simulink model "Output_Feedback"  (R2022b)
settings: Solver=FixedStepAuto  StartTime=0.0  StopTime=10.0  FixedStep=step_size  RelTol=1e-3
undefined symbols (not defined in the file): b, k1, k2, theta_i, x_i, y_i
libraries: simulink_extras x1
settings Model: Creator=Musta  LastModifiedBy=Musta

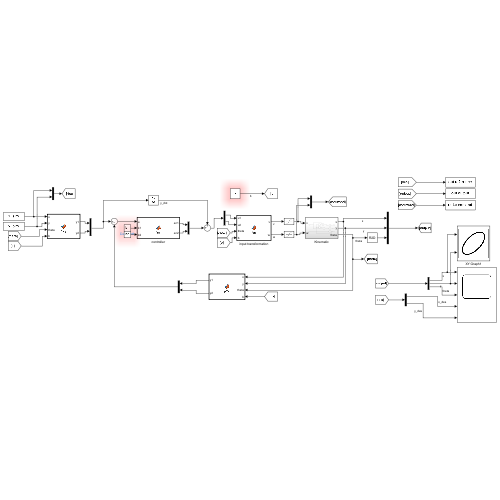
[thumbnail: Simulink's stored preview of the top-level diagram]
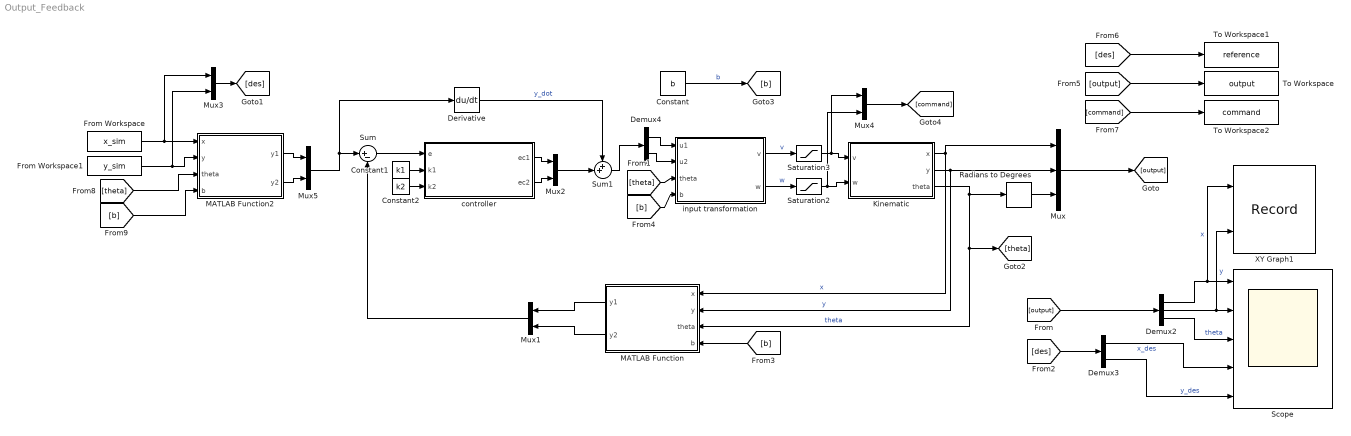
== system Output_Feedback ==
  Constant : Constant  Value=b
  Constant1 : Constant  Value=k1
  Constant2 : Constant  Value=k2
  Demux2 : Demux  Outputs=3
  Demux3 : Demux  Outputs=2
  Demux4 : Demux  Outputs=2
  Derivative : Derivative
  From Workspace : FromWorkspace  VariableName=x_sim
  From Workspace1 : FromWorkspace  VariableName=y_sim
  Kinematic : Subsystem
  MATLAB Function : MATLAB Function  TreatAsAtomicUnit=on
  MATLAB Function2 : MATLAB Function  TreatAsAtomicUnit=on
  Mux : Mux  Inputs=3
  Mux{1..5} (5 alike) : Mux  Inputs=2
  Radians to Degrees : simulink_extras/Transformations/Radians to Degrees
  Saturation2 : Saturate  UpperLimit=2  LowerLimit=-2
  Saturation3 : Saturate  UpperLimit=2  LowerLimit=-2
  Scope : Scope  NumInputPorts=5
  Sum : Sum  Inputs=|+-
  Sum1 : Sum  Inputs=++|
  To Workspace : ToWorkspace  VariableName=output  SaveFormat=Structure With Time  SampleTime=-1
  To Workspace1 : ToWorkspace  VariableName=reference  SaveFormat=Structure With Time  SampleTime=-1
  To Workspace2 : ToWorkspace  VariableName=command  SaveFormat=Structure With Time  SampleTime=-1
  XY Graph1 : Record  FileSettingsInternal="{\"entries\":[{\"content\":{\"excelSettings\":{\"content\":{},\"type\":\"Streamout.ExcelSettings\"}},\"type\":\"Streamout.FileSettingStorage\",\"uuid\":\"0d4e8405-cc65-47cc-850f-a12000fc69a0\"}],\"packageUris\":[\"http://schema.mathworks.com/mf0/streamout_blocks/R2020a\"],\"version\":\"1.0\"}"  Layout=[1 1]  SignalsInternal="{\"entries\":[{\"content\":{\"signals\":[{\"content\":{\"blockPath\":[\"Output_Feedback_MATLAB/XY Graph1\"],\"channel\":[],\"dimensions\":[1],\"domain\":\"Output_Feedback_MATLAB/XY Graph1\",\"lineColor\":\"#a2142f\",\"plots\":[1],\"port\":1,\"sid\":[\"\"],\"signalID\":860,\"signalName\":\"x\"},\"type\":\"RecordBlkView.Signal\",\"uuid\":\"881d64ae-a7b1-402c-b34c-8b1dce287662\"},{\"content\":{\"blockPath\":[\"Output_Feedback_MATLAB/XY Graph1\"],\"channel\":[],\"dimensions\":[1],\"domain\":\"Output_Feedback_MATLAB/XY Graph1\",\"lineColor\":\"#139fff\",\"plots\":[1],\"port\":2,\"sid\":[\"\"],\"signalID\":864,\"signalName\":\"y\"},\"type\":\"RecordBlkView.Signal\",\"uuid\":\"d56edbe0-4863-4ce2-984c-3d6a7468b7cc\"}]},\"type\":\"RecordBlkView.InputSignals\",\"uuid\":\"a5a01336-52e2-4cfc-b20a-f4ad49d08ddd\"}],\"packageUris\":[\"http://schema.mathworks.com/mf0/streamout_blocks/R2020a\"],\"version\":\"1.0\"}"  VisualizationBindings="{\"xyplotplugin\":{\"info\":[{\"series\":[{\"bindingParametersList\":[{\"parameter\":\"X-Axis\",\"signalID\":860,\"signalName\":\"x\"},{\"parameter\":\"Y-Axis\",\"signalID\":864,\"signalName\":\"y\"}],\"seriesID\":40151}],\"subplotID\":1}]}}"  CompatibilityTag=XY
  controller : MATLAB Function  TreatAsAtomicUnit=on
  input transformation : MATLAB Function  TreatAsAtomicUnit=on
  wires:
  [command] -> To Workspace2/1
  Mux4/1 -> [command]
  From Workspace/1 -> Mux3/1, MATLAB Function2/1(x)
  Mux3/1 -> [des]
  [theta] -> MATLAB Function2/3(theta)
  Mux1/1 -> Sum/2
  Radians to Degrees/1 -> Mux/3
  From Workspace1/1 -> Mux3/2, MATLAB Function2/2(y)
  MATLAB Function2/2(y2) -> Mux5/2
  Saturation3/1 -> Kinematic/1(v), Mux4/1
  [des] -> To Workspace1/1
  [des] -> Demux3/1
  [b] -> MATLAB Function/4(b)
  MATLAB Function/2(y2) -> Mux1/2
  MATLAB Function2/1(y1) -> Mux5/1
  [b] -> MATLAB Function2/4(b)
  Derivative/1 -> Sum1/1  "y_dot"
  Mux/1 -> [output]
  Mux5/1 -> Derivative/1, Sum/1
  Demux4/1 -> input transformation/1(u1)
  [theta] -> input transformation/3(theta)
  [output] -> To Workspace/1
  Sum/1 -> controller/1(e)
  Demux4/2 -> input transformation/2(u2)
  Demux2/2 -> XY Graph1/2, Scope/2  "y"
  controller/1(ec1) -> Mux2/1
  [output] -> Demux2/1
  Mux2/1 -> Sum1/2
  Demux2/3 -> Scope/3  "theta"
  Demux3/2 -> Scope/5  "y_des"
  input transformation/1(v) -> Saturation3/1  "v"
  Saturation2/1 -> Kinematic/2(w), Mux4/2
  Constant/1 -> [b]  "b"
  Sum1/1 -> Demux4/1
  Demux2/1 -> XY Graph1/1, Scope/1  "x"
  controller/2(ec2) -> Mux2/2
  MATLAB Function/1(y1) -> Mux1/1
  [b] -> input transformation/4(b)
  Kinematic/3(theta) -> Radians to Degrees/1, [theta], MATLAB Function/3(theta)  "theta"
  input transformation/2(w) -> Saturation2/1  "w"
  Demux3/1 -> Scope/4  "x_des"
  Kinematic/2(y) -> Mux/2, MATLAB Function/2(y)  "y"
  Kinematic/1(x) -> MATLAB Function/1(x), Mux/1  "x"
  Constant2/1 -> controller/3(k2)
  Constant1/1 -> controller/2(k1)

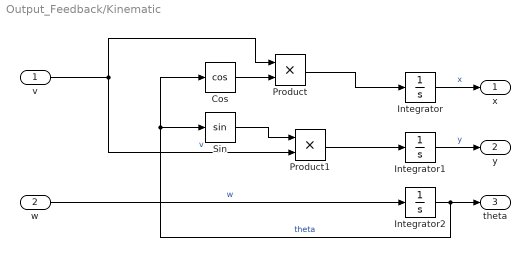
== system Output_Feedback/Kinematic ==
  v : Inport
  w : Inport  Port=2
  Cos : Trigonometry  Operator=cos
  Integrator : Integrator  InitialCondition=x_i
  Integrator1 : Integrator  InitialCondition=y_i
  Integrator2 : Integrator  InitialCondition=theta_i
  Product : Product
  Product1 : Product
  Sin : Trigonometry
  x : Outport
  y : Outport  Port=2
  theta : Outport  Port=3
  wires:
  w/1 -> Integrator2/1  "w"
  v/1 -> Product/1, Product1/2  "v"
  Cos/1 -> Product/2
  Integrator1/1 -> y/1  "y"
  Integrator/1 -> x/1  "x"
  Integrator2/1 -> theta/1, Cos/1, Sin/1  "theta"
  Sin/1 -> Product1/1
  Product/1 -> Integrator/1
  Product1/1 -> Integrator1/1

== matlab function Output_Feedback/MATLAB Function2 ==
  data: x input; y1 output; y input; y2 output; theta input; b input
function [y1,y2] = p2y(x,y,theta,b)

y1 = x + b*cos(theta);
y2 = y + b*sin(theta);

== matlab function Output_Feedback/input transformation ==
  data: u1 input; u2 input; theta input; v output; b input; w output
function [v,w] = fcn(u1, u2, theta, b)

    R = [cos(theta),      sin(theta);
         -sin(theta)/b, cos(theta)/b];
    
    v = cos(theta)*u1 + sin(theta)*u2;
    w = (-sin(theta)/b)*u1 + (cos(theta)/b)*u2;

end

== matlab function Output_Feedback/MATLAB Function ==
  data: x input; y1 output; y input; theta input; b input; y2 output
function [y1,y2] = p2y(x,y,theta,b)

    y1 = x + b*cos(theta);
    y2 = y + b*sin(theta);
    
end

== matlab function Output_Feedback/controller ==
  data: e input; ec1 output; ec2 output; k1 input; k2 input
function [ec1, ec2] = fcn(e, k1, k2)
    
    ec1 = k1*(e(1));
    ec2 = k2*(e(2));
    
end
